simulink model "EPD629_WilliamsJ_AS12"  (R2021b)
settings: Solver=VariableStepAuto  StartTime=0.0  StopTime=45  MaxStep=0.0005  RelTol=1e-3
values from neighbouring files (symbols this model uses):
  AirMassFracO2 = 0.233    [EPD629_HW12_init.m]
  BPVAreaBreakpoints_pct = BPVAreaData_pct    [EPD629_HW12_init.m]
  BPVAreaData_pct = EGRValveAreaData_pct    [EPD629_HW12_init.m]
  BPVPositionBreakpoints_pct = EGRValvePositionBreakpoints_pct    [EPD629_HW12_init.m]
  BPVPositionData_pct = BPVPositionBreakpoints_pct    [EPD629_HW12_init.m]
  BPVWideOpenArea_mm2 = pi * BPVDiameter_mm^2 / 4    (= 7853.98163397)    [EPD629_HW12_init.m]
  CACDischargeCoefficient_frac = 0.7    [EPD629_HW12_init.m]
  CACEffectivenessData_frac = [1 0.95 0.92 0.885 0.87 0.85]    [EPD629_HW12_init.m]
  CACEffectivenessMassFlowBP_gps = [0 50 100 200 300 500]    [EPD629_HW12_init.m]
  CACFlowRestrictionArea_mm2 = 2000    [EPD629_HW12_init.m]
  CACVolume_L = 40    [EPD629_HW12_init.m]
  ClearanceVolumeTotal_L = 8/15    (= 0.533333333333)    [EPD629_HW12_init.m]
  Cp_cmp = 1.004    [EPD629_HW12_init.m]
  Cp_trb = 1.073    [EPD629_HW12_init.m]
  DesiredFuelBreakpoints_mg = 0:20:500    [EPD629_HW12_init.m]
  DischargeCoefficient_frac = 0.7    [EPD629_HW12_init.m]
  EGRCDischargeCoefficient_frac = 0.7    [EPD629_HW12_init.m]
  EGRCEffectivenessData_frac = [1 0.95 0.92 0.885 0.87 0.85]    [EPD629_HW12_init.m]
  EGRCEffectivenessMassFlowBP_gps = [0 50 100 200 300 500]    [EPD629_HW12_init.m]
  EGRCFlowRestrictionArea_mm2 = 500    [EPD629_HW12_init.m]
  EGRCoolerToValveVolume_L = 2    [EPD629_HW12_init.m]
  EGRValveAreaBreakpoints_pct = EGRValveAreaData_pct    [EPD629_HW12_init.m]
  EGRValveAreaData_pct = 100 * EGRValveArea_mm2 / EGRValveWideOpenArea_mm2    [EPD629_HW12_init.m]
  EGRValvePositionBreakpoints_pct = 0:100    [EPD629_HW12_init.m]
  EGRValvePositionData_pct = EGRValvePositionBreakpoints_pct    [EPD629_HW12_init.m]
  EGRValveWideOpenArea_mm2 = pi/4*50^2    (= 1963.49540849)    [EPD629_HW12_init.m]
  EngineDisplacement_L = 8    [EPD629_HW12_init.m]
  EngineSpeedBreakpoints_rpm = 600:200:3000    [EPD629_HW12_init.m]
  ExhaustManifoldGasConstant_kJpkgK = R_trb    (= 0.287)    [EPD629_HW12_init.m]
  ExhaustManifoldVolume_L = 8    [EPD629_HW12_init.m]
  FlowFunctionData_frac = PR.^(1/k_trb) .*      sqrt( 2 * k_trb / (k_trb - 1) .*      (1 - PR.^((k_trb - 1) / k_trb)) )    [EPD629_HW12_init.m]
  IntakeManifoldGasConstant_kJpkgK = Cp_im - Cv_im    (= 0.288)    [EPD629_HW12_init.m]
  IntakeManifoldVolume_L = 8    [EPD629_HW12_init.m]
  k_cmp = Cp_cmp/Cv_cmp    (= 1.40027894003)    [EPD629_HW12_init.m]
  k_trb = Cp_trb/Cv_trb    (= 1.36513994911)    [EPD629_HW12_init.m]
  ManifoldPressureBreakpoints_kPa = 80:20:500    [EPD629_HW12_init.m]
  NumberOfCylinders = 6    [EPD629_HW12_init.m]
  PressureRatioBreakpoints_frac = 0:0.01:1    [EPD629_HW12_init.m]
  R_cmp = Cp_cmp - Cv_cmp    (= 0.287)    [EPD629_HW12_init.m]
  R_trb = Cp_trb - Cv_trb    (= 0.287)    [EPD629_HW12_init.m]
  StoichiometricAFR_frac = 14.7    [EPD629_HW12_init.m]
  TurbineToBPVVolume_L = 10    [EPD629_HW12_init.m]
  TurbochargerInertia_kgm2 = 1e-4    (= 0.0001)    [EPD629_HW12_init.m]
  WastegateAreaData_pct = [0 100]    [EPD629_HW12_init.m]
  WastegateAreaGagePressBreakpoints_kPa = [250 300]    [EPD629_HW12_init.m]
  WastegateWideOpenArea_mm2 = pi/4*20^2    (= 314.159265359)    [EPD629_HW12_init.m]
undefined symbols (not defined in the file or in its folder): APPR_cmp, APPR_trb, ARPM_cmp, ARPM_trb, EFFI_cmp, EFFI_trb, ExhaustTemperatureData_degC, MASS_cmp, MASS_trb, MXRSP_cmp, MXRSP_trb, MXRVOL_cmp, MXRVOL_trb, PMAX_cmp, PMAX_trb, PMIN_cmp, PMIN_trb, ResidualCorrectionFactorData, VolumetricEfficiencyData_frac
libraries: simulink x2
(part 1 of 3)
settings Model: Creator=John  LastModifiedBy=Justin
settings SolverCC: AlgebraicLoopSolver=TrustRegion
settings DebuggingCC: SFMachineParentedDataDiag=warning

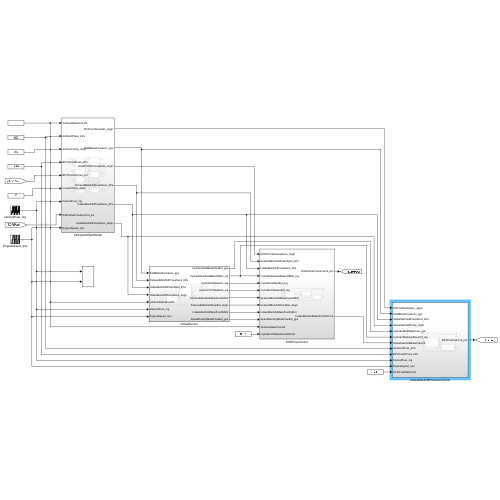
[thumbnail: Simulink's stored preview of the top-level diagram]
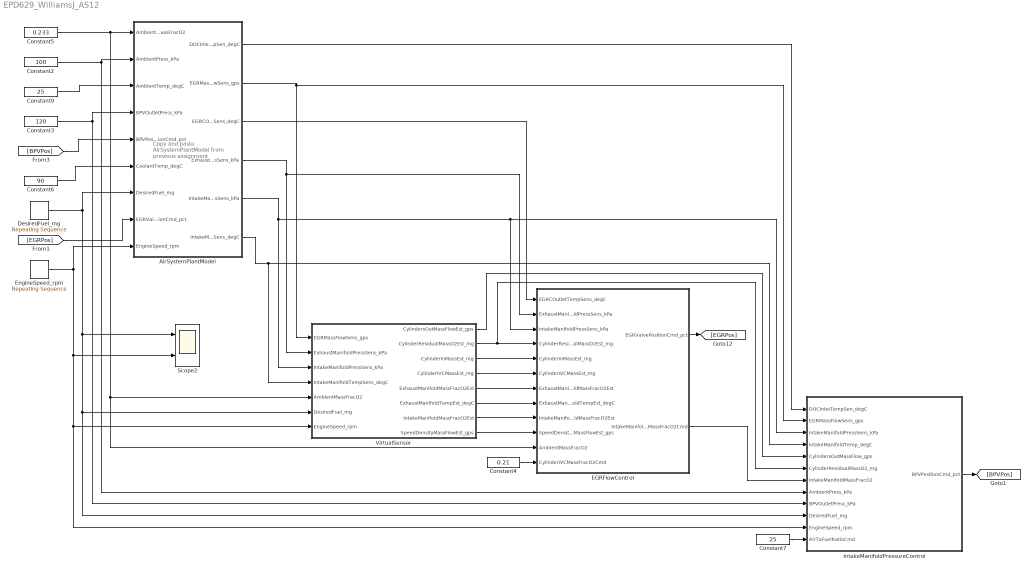
== system EPD629_WilliamsJ_AS12 ==
  note: Copy and paste
      | AirSystemPlantModel
      | from previous assignment
  AirSystemPlantModel : Subsystem
  Constant2 : Constant  Value=100
  Constant3 : Constant  Value=120
  Constant4 : Constant  Value=0.21
  Constant5 : Constant  Value=0.233
  Constant6 : Constant  Value=90
  Constant7 : Constant  Value=25
  Constant9 : Constant  Value=25
  DesiredFuel_mg : simulink/Sources/Repeating Sequence  rep_seq_t="0.25*[0 20 20.1 40 40.1 60    60.1 80 80.1 100 100.1 120    120.1 140 140.1 160 160.1 180]"  rep_seq_y="[40 40 80 80 120 120    70 70 140 140 210 210    90 90 180 180 220 220]"
  EGRFlowControl : Subsystem
  EngineSpeed_rpm : simulink/Sources/Repeating Sequence  rep_seq_t=0.25*[0 60 60.1 120 120.1 180]  rep_seq_y=[1200 1200 1600 1600 2000 2000]
  IntakeManifoldPressureControl : Subsystem
  Scope2 : Scope  NumInputPorts=2
  VirtualSensor : Subsystem
  wires:
  Constant9/1 -> AirSystemPlantModel/3(AmbientTemp_degC)
  Constant6/1 -> AirSystemPlantModel/6(CoolantTemp_degC)
  Constant2/1 -> AirSystemPlantModel/2(AmbientPress_kPa), IntakeManifoldPressureControl/8(AmbientPress_kPa)
  Constant3/1 -> AirSystemPlantModel/4(BPVOutletPress_kPa), IntakeManifoldPressureControl/9(BPVOutletPress_kPa)
  [BPVPos] -> AirSystemPlantModel/5(BPVPositionCmd_pct)
  Constant5/1 -> AirSystemPlantModel/1(AmbientMassFracO2), VirtualSensor/5(AmbientMassFracO2), EGRFlowControl/11(AmbientMassFracO2)
  AirSystemPlantModel/2(EGRMassFlowSens_gps) -> VirtualSensor/1(EGRMassFlowSens_gps), IntakeManifoldPressureControl/2(EGRMassFlowSens_gps)
  AirSystemPlantModel/4(ExhaustManifoldPressSens_kPa) -> VirtualSensor/2(ExhaustManifoldPressSens_kPa), EGRFlowControl/2(ExhaustManifoldPressSens_kPa)
  AirSystemPlantModel/5(IntakeManifoldPressSens_kPa) -> EGRFlowControl/3(IntakeManifoldPressSens_kPa), IntakeManifoldPressureControl/3(IntakeManifoldPressSens_kPa), VirtualSensor/3(IntakeManifoldPressSens_kPa)
  AirSystemPlantModel/6(IntakeManifoldTempSens_degC) -> VirtualSensor/4(IntakeManifoldTempSens_degC), IntakeManifoldPressureControl/4(IntakeManifoldTemp_degC)
  VirtualSensor/5(ExhaustManifoldMassFracO2Est) -> EGRFlowControl/7(ExhaustManifoldMassFracO2Est)
  VirtualSensor/7(IntakeManifoldMassFracO2Est) -> EGRFlowControl/9(IntakeManifoldMassFracO2Est)
  VirtualSensor/3(CylinderInMassEst_mg) -> EGRFlowControl/5(CylinderInMassEst_mg)
  VirtualSensor/4(CylinderIVCMassEst_mg) -> EGRFlowControl/6(CylinderIVCMassEst_mg)
  Constant4/1 -> EGRFlowControl/12(CylinderIVCMassFracO2Cmd)
  DesiredFuel_mg/1 -> AirSystemPlantModel/7(DesiredFuel_mg), IntakeManifoldPressureControl/10(DesiredFuel_mg), VirtualSensor/6(DesiredFuel_mg), Scope2/1
  EngineSpeed_rpm/1 -> AirSystemPlantModel/9(EngineSpeed_rpm), IntakeManifoldPressureControl/11(EngineSpeed_rpm), VirtualSensor/7(EngineSpeed_rpm), Scope2/2
  VirtualSensor/2(CylinderResidualMassO2Est_mg) -> EGRFlowControl/4(CylinderResidualMassO2Est_mg), IntakeManifoldPressureControl/6(CylinderResidualMassO2_mg)
  EGRFlowControl/2(IntakeManifoldMassFracO2Cmd) -> IntakeManifoldPressureControl/7(IntakeManifoldMassFracO2)
  Constant7/1 -> IntakeManifoldPressureControl/12(AirToFuelRatioCmd)
  [EGRPos] -> AirSystemPlantModel/8(EGRValvePositionCmd_pct)
  AirSystemPlantModel/1(DOCInletTempSen_degC) -> IntakeManifoldPressureControl/1(DOCInletTempSen_degC)
  VirtualSensor/8(SpeedDensityMassFlowEst_gps) -> EGRFlowControl/10(SpeedDensityMassFlowEst_gps)
  EGRFlowControl/1(EGRValvePositionCmd_pct) -> [EGRPos]
  AirSystemPlantModel/3(EGRCOutletTempSens_degC) -> EGRFlowControl/1(EGRCOutletTempSens_degC)
  VirtualSensor/6(ExhaustManifoldTempEst_degC) -> EGRFlowControl/8(ExhaustManifoldTempEst_degC)
  IntakeManifoldPressureControl/1(BPVPositionCmd_pct) -> [BPVPos]
  VirtualSensor/1(CylindersOutMassFlowEst_gps) -> IntakeManifoldPressureControl/5(CylindersOutMassFlow_gps)

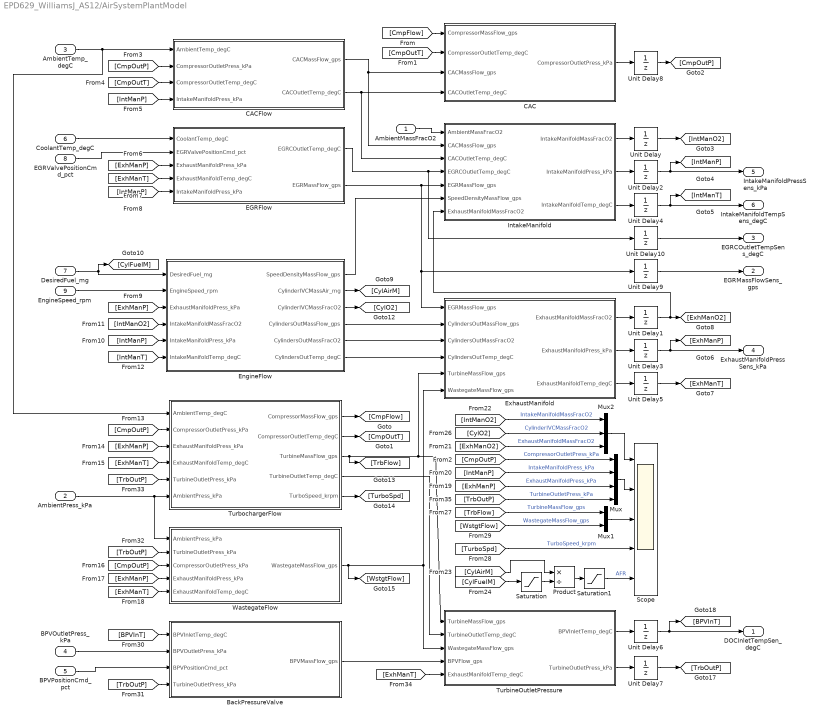
== system EPD629_WilliamsJ_AS12/AirSystemPlantModel ==
  AmbientMassFracO2 : Inport
  AmbientPress_kPa : Inport  Port=2
  AmbientTemp_degC : Inport  Port=3
  BPVOutletPress_kPa : Inport  Port=4
  BPVPositionCmd_pct : Inport  Port=5
  CoolantTemp_degC : Inport  Port=6
  DesiredFuel_mg : Inport  Port=7
  EGRValvePositionCmd_pct : Inport  Port=8
  EngineSpeed_rpm : Inport  Port=9
  BackPressureValve : Subsystem
  CAC : Subsystem
  CACFlow : Subsystem
  EGRFlow : Subsystem
  EngineFlow : Subsystem
  ExhaustManifold : Subsystem
  IntakeManifold : Subsystem
  Mux : Mux
  Mux1 : Mux  Inputs=2
  Mux2 : Mux  Inputs=3
  Product : Product  Inputs=*/
  Saturation : Saturate  UpperLimit=1000  LowerLimit=0.1
  Saturation1 : Saturate  UpperLimit=200  LowerLimit=0
  Scope : Scope  NumInputPorts=5
  TurbineOutletPressure : Subsystem
  TurbochargerFlow : Subsystem
  Unit Delay : UnitDelay  InitialCondition=0.233  SampleTime=-1  HasFrameUpgradeWarning=on
      settings: AttributesFormatString=IC: %<InitialCondition>
  Unit Delay1 : UnitDelay  InitialCondition=0.233  SampleTime=-1  HasFrameUpgradeWarning=on
      settings: AttributesFormatString=IC: %<InitialCondition>
  Unit Delay{4..6,10} (4 alike) : UnitDelay  InitialCondition=25  SampleTime=-1  HasFrameUpgradeWarning=on
      settings: AttributesFormatString=IC: %<InitialCondition>
  Unit Delay{2..3,7..8} (4 alike) : UnitDelay  InitialCondition=100  SampleTime=-1  HasFrameUpgradeWarning=on
      settings: AttributesFormatString=IC: %<InitialCondition>
  Unit Delay9 : UnitDelay  SampleTime=-1  HasFrameUpgradeWarning=on
      settings: AttributesFormatString=IC: %<InitialCondition>
  WastegateFlow : Subsystem
  DOCInletTempSen_degC : Outport
  EGRMassFlowSens_gps : Outport  Port=2
  EGRCOutletTempSens_degC : Outport  Port=3
  ExhaustManifoldPressSens_kPa : Outport  Port=4
  IntakeManifoldPressSens_kPa : Outport  Port=5
  IntakeManifoldTempSens_degC : Outport  Port=6
  wires:
  [IntManT] -> EngineFlow/6(IntakeManifoldTemp_degC)
  AmbientPress_kPa/1 -> WastegateFlow/1(AmbientPress_kPa), TurbochargerFlow/6(AmbientPress_kPa)
  [ExhManO2] -> Mux2/3  "ExhaustManifoldMassFracO2"
  [ExhManP] -> Mux/3  "ExhaustManifoldPress_kPa"
  EGRFlow/2(EGRMassFlow_gps) -> ExhaustManifold/1(EGRMassFlow_gps), Unit Delay9/1, IntakeManifold/5(EGRMassFlow_gps)
  Mux/1 -> Scope/2
  [CmpOutT] -> CAC/2(CompressorOutletTemp_degC)
  [ExhManP] -> EngineFlow/3(ExhaustManifoldPress_kPa)
  AmbientTemp_degC/1 -> TurbochargerFlow/1(AmbientTemp_degC), CACFlow/1(AmbientTemp_degC)
  [TrbFlow] -> Mux1/1  "TurbineMassFlow_gps"
  ExhaustManifold/3(ExhaustManifoldTemp_degC) -> Unit Delay5/1
  CACFlow/1(CACMassFlow_gps) -> IntakeManifold/2(CACMassFlow_gps), CAC/3(CACMassFlow_gps)
  [ExhManP] -> TurbochargerFlow/3(ExhaustManifoldPress_kPa)
  EGRValvePositionCmd_pct/1 -> EGRFlow/2(EGRValvePositionCmd_pct)
  [CmpOutP] -> TurbochargerFlow/2(CompressorOutletPress_kPa)
  TurbochargerFlow/2(CompressorOutletTemp_degC) -> [CmpOutT]
  [TurboSpd] -> Scope/4  "TurboSpeed_krpm"
  [CmpOutP] -> CACFlow/2(CompressorOutletPress_kPa)
  [CmpOutT] -> CACFlow/3(CompressorOutletTemp_degC)
  CACFlow/2(CACOutletTemp_degC) -> CAC/4(CACOutletTemp_degC), IntakeManifold/3(CACOutletTemp_degC)
  [IntManP] -> CACFlow/4(IntakeManifoldPress_kPa)
  [BPVInT] -> BackPressureValve/1(BPVInletTemp_degC)
  EngineSpeed_rpm/1 -> EngineFlow/2(EngineSpeed_rpm)
  WastegateFlow/1(WastegateMassFlow_gps) -> ExhaustManifold/6(WastegateMassFlow_gps), TurbineOutletPressure/3(WastegateMassFlow_gps), [WstgtFlow]
  CAC/1(CompressorOutletPress_kPa) -> Unit Delay8/1
  Mux1/1 -> Scope/3
  TurbochargerFlow/5(TurboSpeed_krpm) -> [TurboSpd]
  TurbochargerFlow/1(CompressorMassFlow_gps) -> [CmpFlow]
  [ExhManT] -> WastegateFlow/5(ExhaustManifoldTemp_degC)
  [IntManO2] -> EngineFlow/4(IntakeManifoldMassFracO2)
  [ExhManP] -> WastegateFlow/4(ExhaustManifoldPress_kPa)
  [CmpFlow] -> CAC/1(CompressorMassFlow_gps)
  [ExhManT] -> TurbochargerFlow/4(ExhaustManifoldTemp_degC)
  DesiredFuel_mg/1 -> [CylFuelM], EngineFlow/1(DesiredFuel_mg)
  [CmpOutP] -> WastegateFlow/3(CompressorOutletPress_kPa)
  TurbochargerFlow/3(TurbineMassFlow_gps) -> [TrbFlow], ExhaustManifold/5(TurbineMassFlow_gps), TurbineOutletPressure/1(TurbineMassFlow_gps)
  [ExhManP] -> EGRFlow/3(ExhaustManifoldPress_kPa)
  IntakeManifold/3(IntakeManifoldTemp_degC) -> Unit Delay4/1
  BackPressureValve/1(BPVMassFlow_gps) -> TurbineOutletPressure/4(BPVFlow_gps)
  [IntManP] -> EGRFlow/5(IntakeManifoldPress_kPa)
  [CmpOutP] -> Mux/1  "CompressorOutletPress_kPa"
  EngineFlow/1(SpeedDensityMassFlow_gps) -> IntakeManifold/6(SpeedDensityMassFlow_gps)
  ExhaustManifold/2(ExhaustManifoldPress_kPa) -> Unit Delay3/1
  IntakeManifold/2(IntakeManifoldPress_kPa) -> Unit Delay2/1
  EGRFlow/1(EGRCOutletTemp_degC) -> Unit Delay10/1, IntakeManifold/4(EGRCOutletTemp_degC)
  Mux2/1 -> Scope/1
  TurbochargerFlow/4(TurbineOutletTemp_degC) -> TurbineOutletPressure/2(TurbineOutletTemp_degC)
  [IntManO2] -> Mux2/1  "IntakeManifoldMassFracO2"
  [IntManP] -> Mux/2  "IntakeManifoldPress_kPa"
  [TrbOutP] -> Mux/4  "TurbineOutletPress_kPa"
  [ExhManT] -> EGRFlow/4(ExhaustManifoldTemp_degC)
  [CylO2] -> Mux2/2  "CylinderIVCMassFracO2"
  [WstgtFlow] -> Mux1/2  "WastegateMassFlow_gps"
  TurbineOutletPressure/1(BPVInletTemp_degC) -> Unit Delay6/1
  [TrbOutP] -> BackPressureValve/4(TurbineOutletPress_kPa)
  TurbineOutletPressure/2(TurbineOutletPress_kPa) -> Unit Delay7/1
  [TrbOutP] -> TurbochargerFlow/5(TurbineOutletPress_kPa)
  [TrbOutP] -> WastegateFlow/2(TurbineOutletPress_kPa)
  [ExhManT] -> TurbineOutletPressure/5(ExhaustManifoldTemp_degC)
  CoolantTemp_degC/1 -> EGRFlow/1(CoolantTemp_degC)
  BPVOutletPress_kPa/1 -> BackPressureValve/2(BPVOutletPress_kPa)
  BPVPositionCmd_pct/1 -> BackPressureValve/3(BPVPositionCmd_pct)
  AmbientMassFracO2/1 -> IntakeManifold/1(AmbientMassFracO2)
  IntakeManifold/1(IntakeManifoldMassFracO2) -> Unit Delay/1
  Unit Delay/1 -> [IntManO2]
  Unit Delay1/1 -> IntakeManifold/7(ExhaustManifoldMassFracO2), [ExhManO2]
  Unit Delay2/1 -> IntakeManifoldPressSens_kPa/1, [IntManP]
  Unit Delay3/1 -> ExhaustManifoldPressSens_kPa/1, [ExhManP]
  Unit Delay4/1 -> IntakeManifoldTempSens_degC/1, [IntManT]
  Unit Delay5/1 -> [ExhManT]
  Unit Delay6/1 -> [BPVInT], DOCInletTempSen_degC/1
  Unit Delay7/1 -> [TrbOutP]
  Unit Delay8/1 -> [CmpOutP]
  Unit Delay9/1 -> EGRMassFlowSens_gps/1
  ExhaustManifold/1(ExhaustManifoldMassFracO2) -> Unit Delay1/1
  Unit Delay10/1 -> EGRCOutletTempSens_degC/1
  Product/1 -> Saturation1/1
  [CylFuelM] -> Saturation/1
  Saturation/1 -> Product/2
  [CylAirM] -> Product/1
  Saturation1/1 -> Scope/5  "AFR"
  [IntManP] -> EngineFlow/5(IntakeManifoldPress_kPa)
  EngineFlow/6(CylindersOutTemp_degC) -> ExhaustManifold/4(CylindersOutTemp_degC)
  EngineFlow/5(CylindersOutMassFracO2) -> ExhaustManifold/3(CylindersOutMassFracO2)
  EngineFlow/4(CylindersOutMassFlow_gps) -> ExhaustManifold/2(CylindersOutMassFlow_gps)
  EngineFlow/2(CylinderIVCMassAir_mg) -> [CylAirM]
  EngineFlow/3(CylinderIVCMassFracO2) -> [CylO2]

== system EPD629_WilliamsJ_AS12/EGRFlowControl ==
  EGRCOutletTempSens_degC : Inport
  ExhaustManifoldPressSens_kPa : Inport  Port=2
  IntakeManifoldPressSens_kPa : Inport  Port=3
  CylinderResidualMassO2Est_mg : Inport  Port=4
  CylinderInMassEst_mg : Inport  Port=5
  CylinderIVCMassEst_mg : Inport  Port=6
  ExhaustManifoldMassFracO2Est : Inport  Port=7
  ExhaustManifoldTempEst_degC : Inport  Port=8
  IntakeManifoldMassFracO2Est : Inport  Port=9
  SpeedDensityMassFlowEst_gps : Inport  Port=10
  AmbientMassFracO2 : Inport  Port=11
  CylinderIVCMassFracO2Cmd : Inport  Port=12
  CoolerOutletPressureCommand : Subsystem
  EGRMassFlowCommand : Subsystem
  EGRValvePositionCommand : Subsystem
  IntakeManifoldMassFractionO2Command : Subsystem
  Mux : Mux  Inputs=2
  Scope2 : Scope  NumInputPorts=4
  EGRValvePositionCmd_pct : Outport
  IntakeManifoldMassFracO2Cmd : Outport  Port=2
  wires:
  CylinderInMassEst_mg/1 -> IntakeManifoldMassFractionO2Command/1(CylinderInMassEst_mg)
  CylinderIVCMassEst_mg/1 -> IntakeManifoldMassFractionO2Command/2(CylinderIVCMassEst_mg)
  CylinderIVCMassFracO2Cmd/1 -> IntakeManifoldMassFractionO2Command/3(CylinderIVCMassFracO2Cmd)
  EGRValvePositionCommand/1(EGRValvePositionCmd_pct) -> EGRMassFlowCommand/6(EGRValvePositionCmd_pct), Scope2/4, EGRValvePositionCmd_pct/1
  IntakeManifoldMassFracO2Est/1 -> Mux/2, EGRMassFlowCommand/2(IntakeManifoldMassFracO2Est)
  AmbientMassFracO2/1 -> EGRMassFlowCommand/3(AmbientMassFracO2)
  SpeedDensityMassFlowEst_gps/1 -> EGRMassFlowCommand/5(SpeedDensityMassFlowEst_gps)
  ExhaustManifoldMassFracO2Est/1 -> EGRMassFlowCommand/4(ExhaustManifoldMassFracO2Est)
  IntakeManifoldMassFractionO2Command/1(IntakeManifoldMassFracO2Cmd) -> IntakeManifoldMassFracO2Cmd/1, EGRMassFlowCommand/1(IntakeManifoldMassFracO2Cmd), Mux/1
  CylinderResidualMassO2Est_mg/1 -> IntakeManifoldMassFractionO2Command/4(CylinderResidualMassO2Est_mg)
  EGRCOutletTempSens_degC/1 -> EGRValvePositionCommand/2(EGRCOutletTempSens_degC), CoolerOutletPressureCommand/3(EGRCOutletTempSens_degC)
  ExhaustManifoldPressSens_kPa/1 -> CoolerOutletPressureCommand/1(ExhaustManifoldPressSens_kPa)
  IntakeManifoldPressSens_kPa/1 -> EGRValvePositionCommand/4(IntakeManifoldPressSens_kPa)
  CoolerOutletPressureCommand/1(EGRCOutletPressCmd_kPa) -> EGRValvePositionCommand/1(EGRCOutletPressCmd_kPa), Scope2/3
  EGRMassFlowCommand/1(EGRMassFlowCmd_gps) -> Scope2/2, CoolerOutletPressureCommand/4(EGRMassFlowCmd_gps), EGRValvePositionCommand/3(EGRMassFlowCmd_gps)
  ExhaustManifoldTempEst_degC/1 -> CoolerOutletPressureCommand/2(ExhaustManifoldTempEst_degC)
  Mux/1 -> Scope2/1

== system EPD629_WilliamsJ_AS12/IntakeManifoldPressureControl ==
  DOCInletTempSen_degC : Inport
  EGRMassFlowSens_gps : Inport  Port=2
  IntakeManifoldPressSens_kPa : Inport  Port=3
  IntakeManifoldTemp_degC : Inport  Port=4
  CylindersOutMassFlow_gps : Inport  Port=5
  CylinderResidualMassO2_mg : Inport  Port=6
  IntakeManifoldMassFracO2 : Inport  Port=7
  AmbientPress_kPa : Inport  Port=8
  BPVOutletPress_kPa : Inport  Port=9
  DesiredFuel_mg : Inport  Port=10
  EngineSpeed_rpm : Inport  Port=11
  AirToFuelRatioCmd : Inport  Port=12
  BPVInletPressureCommand : Subsystem
  BPVPositionCommand : Subsystem
  IntakeManifoldPressureCommand : Subsystem
  Mux : Mux  Inputs=2
  Scope2 : Scope  NumInputPorts=3
  BPVPositionCmd_pct : Outport
  wires:
  CylindersOutMassFlow_gps/1 -> BPVInletPressureCommand/4(CylindersOutMassFlow_gps)
  EGRMassFlowSens_gps/1 -> BPVInletPressureCommand/5(EGRMassFlowSens_gps)
  IntakeManifoldPressSens_kPa/1 -> Mux/2, BPVInletPressureCommand/3(IntakeManifoldPressSens_kPa)
  BPVInletPressureCommand/1(BPVMassFlowCmd_gps) -> BPVPositionCommand/1(BPVMassFlowCmd_gps)
  BPVInletPressureCommand/2(BPVInletPressCmd_kPa) -> Scope2/2, BPVPositionCommand/2(BPVInletPressCmd_kPa)
  IntakeManifoldTemp_degC/1 -> IntakeManifoldPressureCommand/1(IntakeManifoldTemp_degC)
  CylinderResidualMassO2_mg/1 -> IntakeManifoldPressureCommand/2(CylinderResidualMassO2_mg)
  IntakeManifoldMassFracO2/1 -> IntakeManifoldPressureCommand/3(IntakeManifoldMassFracO2)
  DesiredFuel_mg/1 -> IntakeManifoldPressureCommand/4(DesiredFuel_mg)
  EngineSpeed_rpm/1 -> IntakeManifoldPressureCommand/5(EngineSpeed_rpm)
  AirToFuelRatioCmd/1 -> IntakeManifoldPressureCommand/6(AirToFuelRatioCmd)
  IntakeManifoldPressureCommand/1(IntakeManifoldPressCmd_kPa) -> BPVInletPressureCommand/1(IntakeManifoldPressCmd_kPa), Mux/1
  BPVPositionCommand/1(BPVPositionCmd_pct) -> BPVInletPressureCommand/6(BPVPositionCmd_pct), Scope2/3, BPVPositionCmd_pct/1
  DOCInletTempSen_degC/1 -> BPVPositionCommand/4(DOCInletTempSen_degC)
  BPVOutletPress_kPa/1 -> BPVPositionCommand/3(BPVOutletPress_kPa)
  Mux/1 -> Scope2/1
  AmbientPress_kPa/1 -> BPVInletPressureCommand/2(AmbientPress_kPa), IntakeManifoldPressureCommand/7(AmbientPress_kPa)

== system EPD629_WilliamsJ_AS12/VirtualSensor ==
  EGRMassFlowSens_gps : Inport
  ExhaustManifoldPressSens_kPa : Inport  Port=2
  IntakeManifoldPressSens_kPa : Inport  Port=3
  IntakeManifoldTempSens_degC : Inport  Port=4
  AmbientMassFracO2 : Inport  Port=5
  DesiredFuel_mg : Inport  Port=6
  EngineSpeed_rpm : Inport  Port=7
  EngineFlow : Subsystem
  ExhaustManifoldMassFraction : Subsystem
  IntakeManifoldMassFraction : Subsystem
  Terminator : Terminator
  Terminator1 : Terminator
  Terminator2 : Terminator
  CylindersOutMassFlowEst_gps : Outport
  CylinderResidualMassO2Est_mg : Outport  Port=2
  CylinderInMassEst_mg : Outport  Port=3
  CylinderIVCMassEst_mg : Outport  Port=4
  ExhaustManifoldMassFracO2Est : Outport  Port=5
  ExhaustManifoldTempEst_degC : Outport  Port=6
  IntakeManifoldMassFracO2Est : Outport  Port=7
  SpeedDensityMassFlowEst_gps : Outport  Port=8
  wires:
  EngineFlow/10(SpeedDensityMassFlow_gps) -> SpeedDensityMassFlowEst_gps/1, IntakeManifoldMassFraction/6(SpeedDensityMassFlowEst_gps)
  DesiredFuel_mg/1 -> EngineFlow/2(DesiredFuel_mg)
  EngineSpeed_rpm/1 -> EngineFlow/3(EngineSpeed_rpm)
  AmbientMassFracO2/1 -> IntakeManifoldMassFraction/3(AmbientMassFracO2)
  EGRMassFlowSens_gps/1 -> IntakeManifoldMassFraction/4(EGRMassFlowSens_gps)
  IntakeManifoldMassFraction/1(IntakeManifoldMassFracO2Est) -> EngineFlow/6(IntakeManifoldMassFracO2), IntakeManifoldMassFracO2Est/1
  IntakeManifoldPressSens_kPa/1 -> IntakeManifoldMassFraction/1(IntakeManifoldPressSens_kPa), EngineFlow/4(IntakeManifoldPress_kPa)
  IntakeManifoldTempSens_degC/1 -> IntakeManifoldMassFraction/2(IntakeManifoldTemp_degC), EngineFlow/5(IntakeManifoldTemp_degC)
  ExhaustManifoldPressSens_kPa/1 -> EngineFlow/1(ExhaustManifoldPress_kPa), ExhaustManifoldMassFraction/1(ExhaustManifoldPressSens_kPa)
  EngineFlow/1(CylindersOutMassFlow_gps) -> ExhaustManifoldMassFraction/2(CylindersOutMassFlowEst_gps), CylindersOutMassFlowEst_gps/1
  EngineFlow/3(CylindersOutTemp_degC) -> ExhaustManifoldTempEst_degC/1, ExhaustManifoldMassFraction/4(CylindersOutTempEst_degC)
  EngineFlow/2(CylindersOutMassFracO2) -> ExhaustManifoldMassFraction/3(CylindersOutMassFracO2Est)
  ExhaustManifoldMassFraction/1(ExhaustManifoldMassFracO2Est) -> IntakeManifoldMassFraction/5(ExhaustManifoldMassFracO2Est), ExhaustManifoldMassFracO2Est/1
  EngineFlow/4(CylinderInMass_mg) -> CylinderInMassEst_mg/1
  EngineFlow/6(CylinderIVCMassAir_mg) -> Terminator/1
  EngineFlow/7(CylinderIVCMassFracO2) -> Terminator1/1
  EngineFlow/5(CylinderIVCMass_mg) -> CylinderIVCMassEst_mg/1
  EngineFlow/9(CylinderResidualMassO2_mg) -> CylinderResidualMassO2Est_mg/1
  EngineFlow/8(CylinderResidualMass_mg) -> Terminator2/1

== system EPD629_WilliamsJ_AS12/AirSystemPlantModel/BackPressureValve ==
  note: K
  note: g*m/s^2/mm^2
  note: m^2/s^2
  note: k kg*m/s^2/m^2
  note: N*m/kg
  note: m/s
  note: kPa
  BPVInletTemp_degC : Inport
  BPVOutletPress_kPa : Inport  Port=2
  BPVPositionCmd_pct : Inport  Port=3
  TurbineOutletPress_kPa : Inport  Port=4
  Add1 : Sum
  BPVAreaData_pct Table : Lookup_n-D  NumberOfTableDimensions=1  BreakpointsForDimension1=BPVPositionBreakpoints_pct  Table=BPVAreaData_pct  ExtrapMethod=Clip  UseLastTableValue=on  InternalRulePriority=Speed  RndMeth=Simplest  InputSameDT=on
  Constant : Constant  Value=273.15
  Constant1 : Constant  Value=DischargeCoefficient_frac
  Constant2 : Constant
  Constant3 : Constant  Value=ExhaustManifoldGasConstant_kJpkgK
  Constant5 : Constant  Value=BPVWideOpenArea_mm2
  Constant6 : Constant  Value=100
  FlowFunctionData_frac Table : Lookup_n-D  NumberOfTableDimensions=1  BreakpointsForDimension1=PressureRatioBreakpoints_frac  Table=FlowFunctionData_frac  ExtrapMethod=Clip  UseLastTableValue=on  InternalRulePriority=Speed  RndMeth=Simplest  InputSameDT=on
  Math Function : Math  Operator=sqrt  SignedPower=on  SaturateOnIntegerOverflow=on
  Max2 : MinMax  Function=max  Inputs=2
  Product : Product  Inputs=**/
  Product1 : Product  Inputs=****/  SaturateOnIntegerOverflow=on  OutDataTypeStr=Inherit: Same as first input
  Product2 : Product  Inputs=*/  SaturateOnIntegerOverflow=on  OutDataTypeStr=Inherit: Same as first input
  Product3 : Product  SaturateOnIntegerOverflow=on  OutDataTypeStr=Inherit: Same as first input
  Transfer Fcn : TransferFcn  Denominator=[0.05 1]
  kJ/(kg*K) to J/(kg*K) : Gain  Gain=1000
  BPVMassFlow_gps : Outport
  wires:
  Add1/1 -> Max2/1
  Constant/1 -> Add1/2
  Constant2/1 -> Max2/2
  BPVInletTemp_degC/1 -> Add1/1
  BPVPositionCmd_pct/1 -> Transfer Fcn/1
  Product/1 -> Product1/1  "BPVArea_mm2"
  Constant5/1 -> Product/2
  Constant6/1 -> Product/3
  Product3/1 -> Math Function/1
  Math Function/1 -> Product1/5
  Max2/1 -> Product3/2
  kJ/(kg*K) to J/(kg*K)/1 -> Product3/1
  Constant3/1 -> kJ/(kg*K) to J/(kg*K)/1
  Constant1/1 -> Product1/2
  Product2/1 -> FlowFunctionData_frac Table/1  "BPVPressureRatio_frac"
  FlowFunctionData_frac Table/1 -> Product1/3
  BPVAreaData_pct Table/1 -> Product/1  "BPVArea_pct"
  TurbineOutletPress_kPa/1 -> Product2/2, Product1/4
  Product1/1 -> BPVMassFlow_gps/1
  BPVOutletPress_kPa/1 -> Product2/1
  Transfer Fcn/1 -> BPVAreaData_pct Table/1

== system EPD629_WilliamsJ_AS12/AirSystemPlantModel/CAC ==
  note: dm/dt
  note: dP/dt
  CompressorMassFlow_gps : Inport
  CompressorOutletTemp_degC : Inport  Port=2
  CACMassFlow_gps : Inport  Port=3
  CACOutletTemp_degC : Inport  Port=4
  Add : Sum  Inputs=+-
  Add1 : Sum  Inputs=2
  Add2 : Sum
  Constant : Constant  Value=273.15
  Constant2 : Constant  Value=IntakeManifoldGasConstant_kJpkgK
  Constant3 : Constant  Value=CACVolume_L
  Gain : Gain  Gain=0.5
  Integrator3 : Integrator  InitialCondition=100  LimitOutput=on  UpperSaturationLimit=1000  LowerSaturationLimit=10
      settings: AttributesFormatString=|
      | Max: %<UpperSaturationLimit>
      | Min: %<LowerSaturationLimit>
      | IC: %<InitialCondition>
  Product1 : Product  Inputs=***/  RndMeth=Zero
  Saturation : Saturate  UpperLimit=1000  LowerLimit=-100
      settings: AttributesFormatString=|
      | Max: %<UpperLimit>
      | Min: %<LowerLimit>
  CompressorOutletPress_kPa : Outport
  wires:
  Constant3/1 -> Product1/4
  Constant2/1 -> Product1/2
  CACMassFlow_gps/1 -> Add/2
  CompressorMassFlow_gps/1 -> Add/1
  Add/1 -> Product1/1
  CompressorOutletTemp_degC/1 -> Add1/1
  CACOutletTemp_degC/1 -> Add1/2
  Add1/1 -> Gain/1
  Constant/1 -> Add2/2
  Gain/1 -> Saturation/1
  Add2/1 -> Product1/3
  Integrator3/1 -> CompressorOutletPress_kPa/1
  Product1/1 -> Integrator3/1
  Saturation/1 -> Add2/1

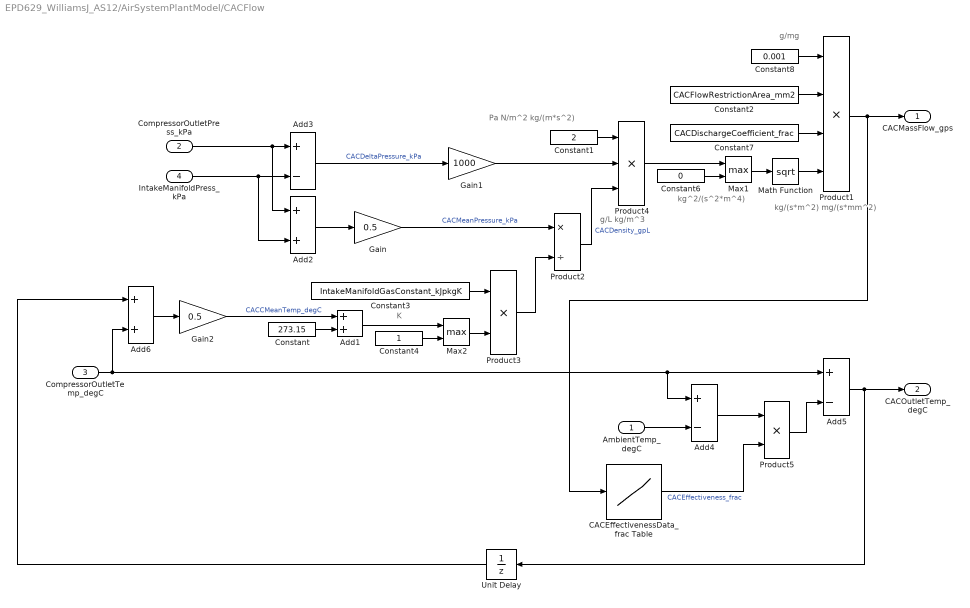
== system EPD629_WilliamsJ_AS12/AirSystemPlantModel/CACFlow ==
  note: g/mg
  note: g/L
      | kg/m^3
  note: kg^2/(s^2*m^4)
  note: Pa
      | N/m^2
      | kg/(m*s^2)
  note: K
  note: kg/(s*m^2)
      | mg/(s*mm^2)
  AmbientTemp_degC : Inport
  CompressorOutletPress_kPa : Inport  Port=2
  CompressorOutletTemp_degC : Inport  Port=3
  IntakeManifoldPress_kPa : Inport  Port=4
  Add1 : Sum
  Add2 : Sum  Inputs=2
  Add3 : Sum  Inputs=+-
  Add4 : Sum  Inputs=+-
  Add5 : Sum  Inputs=+-
  Add6 : Sum  Inputs=2
  CACEffectivenessData_frac Table : Lookup_n-D  NumberOfTableDimensions=1  BreakpointsForDimension1=CACEffectivenessMassFlowBP_gps  Table=CACEffectivenessData_frac  ExtrapMethod=Clip  UseLastTableValue=on  InternalRulePriority=Speed  RndMeth=Simplest  InputSameDT=on
  Constant : Constant  Value=273.15
  Constant1 : Constant  Value=2
  Constant2 : Constant  Value=CACFlowRestrictionArea_mm2
  Constant3 : Constant  Value=IntakeManifoldGasConstant_kJpkgK
  Constant4 : Constant
  Constant6 : Constant  Value=0
  Constant7 : Constant  Value=CACDischargeCoefficient_frac
  Constant8 : Constant  Value=0.001
  Gain : Gain  Gain=0.5
  Gain1 : Gain  Gain=1000
  Gain2 : Gain  Gain=0.5
  Math Function : Math  Operator=sqrt  SignedPower=on  SaturateOnIntegerOverflow=on
  Max1 : MinMax  Function=max  Inputs=2
  Max2 : MinMax  Function=max  Inputs=2
  Product1 : Product  Inputs=4  SaturateOnIntegerOverflow=on  OutDataTypeStr=Inherit: Same as first input
  Product2 : Product  Inputs=*/  SaturateOnIntegerOverflow=on  OutDataTypeStr=Inherit: Same as first input
  Product3 : Product  SaturateOnIntegerOverflow=on  OutDataTypeStr=Inherit: Same as first input
  Product4 : Product  Inputs=3  SaturateOnIntegerOverflow=on  OutDataTypeStr=Inherit: Same as first input
  Product5 : Product  SaturateOnIntegerOverflow=on  OutDataTypeStr=Inherit: Same as first input
  Unit Delay : UnitDelay  InitialCondition=100  SampleTime=-1  HasFrameUpgradeWarning=on
      settings: AttributesFormatString=IC: %<InitialCondition>
  CACMassFlow_gps : Outport
  CACOutletTemp_degC : Outport  Port=2
  wires:
  Constant2/1 -> Product1/2
  Constant3/1 -> Product3/1
  IntakeManifoldPress_kPa/1 -> Add3/2, Add2/2
  Add1/1 -> Max2/1
  Constant/1 -> Add1/2
  Max2/1 -> Product3/2
  Constant4/1 -> Max2/2
  Add5/1 -> Unit Delay/1, CACOutletTemp_degC/1
  Add2/1 -> Gain/1
  Gain/1 -> Product2/1  "CACMeanPressure_kPa"
  Product3/1 -> Product2/2
  Product2/1 -> Product4/3  "CACDensity_gpL"
  Constant1/1 -> Product4/1
  Constant6/1 -> Max1/2
  Product4/1 -> Max1/1
  Max1/1 -> Math Function/1
  Math Function/1 -> Product1/4
  Constant7/1 -> Product1/3
  Gain1/1 -> Product4/2
  Constant8/1 -> Product1/1
  Product1/1 -> CACEffectivenessData_frac Table/1, CACMassFlow_gps/1
  Add3/1 -> Gain1/1  "CACDeltaPressure_kPa"
  CompressorOutletPress_kPa/1 -> Add3/1, Add2/1
  Add4/1 -> Product5/1
  Product5/1 -> Add5/2
  CompressorOutletTemp_degC/1 -> Add6/2, Add4/1, Add5/1
  AmbientTemp_degC/1 -> Add4/2
  CACEffectivenessData_frac Table/1 -> Product5/2  "CACEffectiveness_frac"
  Add6/1 -> Gain2/1
  Gain2/1 -> Add1/1  "CACCMeanTemp_degC"
  Unit Delay/1 -> Add6/1

== system EPD629_WilliamsJ_AS12/AirSystemPlantModel/EGRFlow ==
  CoolantTemp_degC : Inport
  EGRValvePositionCmd_pct : Inport  Port=2
  ExhaustManifoldPress_kPa : Inport  Port=3
  ExhaustManifoldTemp_degC : Inport  Port=4
  IntakeManifoldPress_kPa : Inport  Port=5
  EGRCooler : Subsystem
  EGRCoolerOutletPressure : Subsystem
  EGRCoolerOutletTemperature : Subsystem
  EGRValve : Subsystem
  Unit Delay : UnitDelay  InitialCondition=100  SampleTime=-1  HasFrameUpgradeWarning=on
      settings: AttributesFormatString=IC: %<InitialCondition>
  EGRCOutletTemp_degC : Outport
  EGRMassFlow_gps : Outport  Port=2
  wires:
  ExhaustManifoldTemp_degC/1 -> EGRCoolerOutletTemperature/2(ExhaustManifoldTemp_degC), EGRCooler/2(ExhaustManifoldTemp_degC)
  EGRValvePositionCmd_pct/1 -> EGRValve/2(EGRValvePositionCmd_pct)
  CoolantTemp_degC/1 -> EGRCoolerOutletTemperature/3(CoolantTemp_degC)
  EGRCoolerOutletTemperature/1(EGRCOutletTemp_degC) -> EGRCoolerOutletPressure/3(EGRCOutletTemp_degC), Unit Delay/1, EGRCOutletTemp_degC/1
  IntakeManifoldPress_kPa/1 -> EGRValve/1(IntakeManifoldPress_kPa)
  ExhaustManifoldPress_kPa/1 -> EGRCooler/1(ExhaustManifoldPress_kPa)
  EGRValve/1(EGRValveMassFlow_gps) -> EGRCoolerOutletPressure/2(EGRValveMassFlow_gps), EGRCoolerOutletTemperature/1(EGRMassFlow_gps), EGRMassFlow_gps/1
  EGRCooler/1(EGRCoolerMassFlow_gps) -> EGRCoolerOutletPressure/1(EGRCoolerMassFlow_gps)
  Unit Delay/1 -> EGRCooler/4(EGRCOutletTemp_degC), EGRValve/4(EGRCOutletTemp_degC)
  EGRCoolerOutletPressure/1(EGRCOutletPress_kPa) -> EGRCooler/3(EGRCOutletPress_kPa), EGRValve/3(EGRCOutletPress_kPa)

== system EPD629_WilliamsJ_AS12/AirSystemPlantModel/EngineFlow ==
  DesiredFuel_mg : Inport
  EngineSpeed_rpm : Inport  Port=2
  ExhaustManifoldPress_kPa : Inport  Port=3
  IntakeManifoldMassFracO2 : Inport  Port=4
  IntakeManifoldPress_kPa : Inport  Port=5
  IntakeManifoldTemp_degC : Inport  Port=6
  CylinderEVO : Subsystem
  CylinderIVC : Subsystem
  ExhaustTempAndResidualMass : Subsystem
  SpeedDensityMassFlow : Subsystem
  Terminator : Terminator
  Unit Delay : UnitDelay  SampleTime=-1  HasFrameUpgradeWarning=on
      settings: AttributesFormatString=IC: %<InitialCondition>
  Unit Delay1 : UnitDelay  SampleTime=-1  HasFrameUpgradeWarning=on
      settings: AttributesFormatString=IC: %<InitialCondition>
  SpeedDensityMassFlow_gps : Outport
  CylinderIVCMassAir_mg : Outport  Port=2
  CylinderIVCMassFracO2 : Outport  Port=3
  CylindersOutMassFlow_gps : Outport  Port=4
  CylindersOutMassFracO2 : Outport  Port=5
  CylindersOutTemp_degC : Outport  Port=6
  wires:
  CylinderIVC/2(CylinderIVCMassFracO2) -> CylinderIVCMassFracO2/1
  Unit Delay1/1 -> ExhaustTempAndResidualMass/3(CombustionMassFuel_mg)
  CylinderEVO/3(CombustionMassFuel_mg) -> Unit Delay1/1
  Unit Delay/1 -> CylinderIVC/4(CylindersOutMassFracO2)
  CylinderIVC/4(CylinderIVCMass_mg) -> CylinderEVO/2(CylinderIVCMass_mg)
  CylinderEVO/1(CylindersOutMassFlow_gps) -> CylindersOutMassFlow_gps/1
  CylinderEVO/2(CylindersOutMassFracO2) -> CylindersOutMassFracO2/1, Unit Delay/1
  DesiredFuel_mg/1 -> CylinderEVO/5(DesiredFuel_mg)
  CylinderIVC/3(CylinderIVCMassAir_mg) -> CylinderIVCMassAir_mg/1, CylinderEVO/1(CylinderIVCMassAir_mg)
  IntakeManifoldMassFracO2/1 -> CylinderIVC/2(IntakeManifoldMassFracO2)
  SpeedDensityMassFlow/2(CylinderInMass_mg) -> CylinderIVC/1(CylinderInMass_mg)
  ExhaustTempAndResidualMass/1(CylinderResidualMass_mg) -> CylinderEVO/4(CylinderResidualMass_mg), CylinderIVC/3(CylinderResidualMass_mg)
  ExhaustTempAndResidualMass/2(CylindersOutTemp_degC) -> CylindersOutTemp_degC/1
  ExhaustManifoldPress_kPa/1 -> ExhaustTempAndResidualMass/2(ExhaustManifoldPress_kPa)
  IntakeManifoldTemp_degC/1 -> SpeedDensityMassFlow/2(IntakeManifoldTemp_degC)
  IntakeManifoldPress_kPa/1 -> SpeedDensityMassFlow/1(IntakeManifoldPress_kPa)
  EngineSpeed_rpm/1 -> SpeedDensityMassFlow/3(EngineSpeed_rpm), ExhaustTempAndResidualMass/1(EngineSpeed_rpm), CylinderEVO/3(EngineSpeed_rpm)
  SpeedDensityMassFlow/1(SpeedDensityMassFlow_gps) -> SpeedDensityMassFlow_gps/1
  CylinderIVC/1(CylinderResidualMassO2_mg) -> Terminator/1

== system EPD629_WilliamsJ_AS12/AirSystemPlantModel/ExhaustManifold ==
  note: dmO2/dt
  note: dm/dt
  EGRMassFlow_gps : Inport
  CylindersOutMassFlow_gps : Inport  Port=2
  CylindersOutMassFracO2 : Inport  Port=3
  CylindersOutTemp_degC : Inport  Port=4
  TurbineMassFlow_gps : Inport  Port=5
  WastegateMassFlow_gps : Inport  Port=6
  Add : Sum  Inputs=+-
  Add1 : Sum  Inputs=3
  Add2 : Sum  Inputs=+-
  Add7 : Sum
  Constant7 : Constant  Value=273.15
  Constant8 : Constant  Value=ExhaustManifoldGasConstant_kJpkgK
  Constant9 : Constant  Value=ExhaustManifoldVolume_L
  Integrator1 : Integrator  LimitOutput=on  UpperSaturationLimit=1000  LowerSaturationLimit=0
      settings: AttributesFormatString=|
      | Max: %<UpperSaturationLimit>
      | Min: %<LowerSaturationLimit>
      | IC: %<InitialCondition>
  Integrator3 : Integrator  InitialCondition=10  LimitOutput=on  UpperSaturationLimit=1000  LowerSaturationLimit=1
      settings: AttributesFormatString=|
      | Max: %<UpperSaturationLimit>
      | Min: %<LowerSaturationLimit>
      | IC: %<InitialCondition>
  Product1 : Product  RndMeth=Zero
  Product11 : Product  Inputs=**/  RndMeth=Zero
  Product4 : Product  RndMeth=Zero
  Product6 : Product  RndMeth=Zero
  Product7 : Product  Inputs=*/  RndMeth=Zero
  Saturation : Saturate  UpperLimit=1000  LowerLimit=-100
      settings: AttributesFormatString=|
      | Max: %<UpperLimit>
      | Min: %<LowerLimit>
  Transfer Fcn : TransferFcn  Denominator=[0.05 1]
  ExhaustManifoldMassFracO2 : Outport
  ExhaustManifoldPress_kPa : Outport  Port=2
  ExhaustManifoldTemp_degC : Outport  Port=3
  wires:
  Integrator1/1 -> Product7/1  "ExhaustManifoldMassO2_g"
  Add2/1 -> Integrator1/1
  Product11/1 -> Product1/2
  Constant8/1 -> Product11/1
  Add7/1 -> Product11/2
  Constant9/1 -> Product11/3
  Add/1 -> Integrator3/1
  Constant7/1 -> Add7/2
  Product7/1 -> ExhaustManifoldMassFracO2/1, Product6/2
  Saturation/1 -> Transfer Fcn/1
  Product6/1 -> Add2/2
  Product4/1 -> Add2/1
  CylindersOutMassFracO2/1 -> Product4/2
  CylindersOutTemp_degC/1 -> Saturation/1
  EGRMassFlow_gps/1 -> Add1/1
  TurbineMassFlow_gps/1 -> Add1/2
  WastegateMassFlow_gps/1 -> Add1/3
  Add1/1 -> Product6/1, Add/2
  Integrator3/1 -> Product1/1, Product7/2
  Product1/1 -> ExhaustManifoldPress_kPa/1
  Transfer Fcn/1 -> ExhaustManifoldTemp_degC/1, Add7/1
  CylindersOutMassFlow_gps/1 -> Product4/1, Add/1

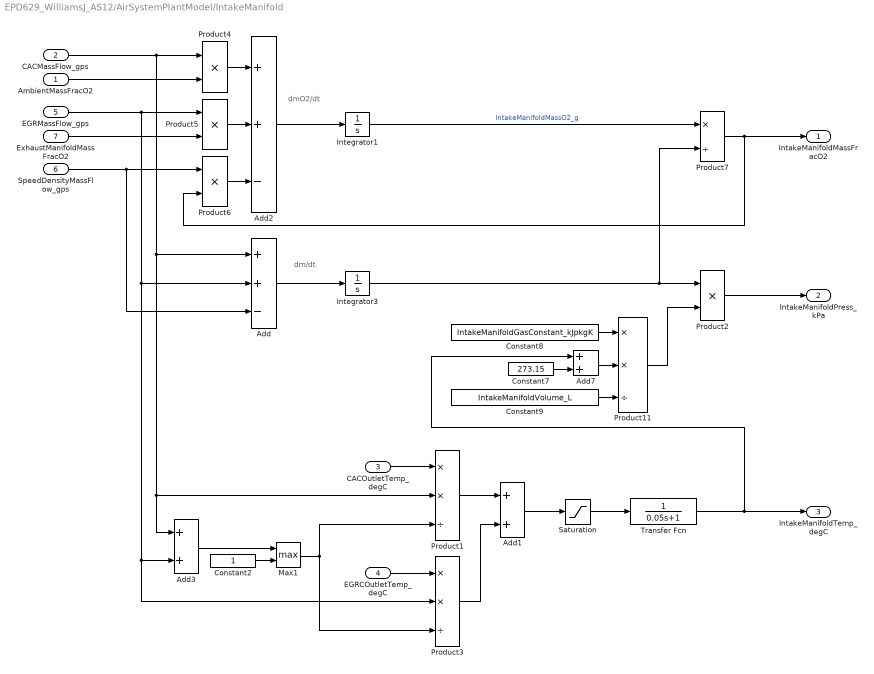
== system EPD629_WilliamsJ_AS12/AirSystemPlantModel/IntakeManifold ==
  note: dm/dt
  note: dmO2/dt
  AmbientMassFracO2 : Inport
  CACMassFlow_gps : Inport  Port=2
  CACOutletTemp_degC : Inport  Port=3
  EGRCOutletTemp_degC : Inport  Port=4
  EGRMassFlow_gps : Inport  Port=5
  SpeedDensityMassFlow_gps : Inport  Port=6
  ExhaustManifoldMassFracO2 : Inport  Port=7
  Add : Sum  Inputs=++-
  Add1 : Sum  Inputs=2
  Add2 : Sum  Inputs=++-
  Add3 : Sum  Inputs=2
  Add7 : Sum
  Constant2 : Constant
  Constant7 : Constant  Value=273.15
  Constant8 : Constant  Value=IntakeManifoldGasConstant_kJpkgK
  Constant9 : Constant  Value=IntakeManifoldVolume_L
  Integrator1 : Integrator  LimitOutput=on  UpperSaturationLimit=1000  LowerSaturationLimit=0
      settings: AttributesFormatString=|
      | Max: %<UpperSaturationLimit>
      | Min: %<LowerSaturationLimit>
      | IC: %<InitialCondition>
  Integrator3 : Integrator  InitialCondition=10  LimitOutput=on  UpperSaturationLimit=1000  LowerSaturationLimit=1
      settings: AttributesFormatString=|
      | Max: %<UpperSaturationLimit>
      | Min: %<LowerSaturationLimit>
      | IC: %<InitialCondition>
  Max1 : MinMax  Function=max  Inputs=2
  Product1 : Product  Inputs=**/  RndMeth=Zero
  Product11 : Product  Inputs=**/  RndMeth=Zero
  Product{2,4..6} (4 alike) : Product  RndMeth=Zero
  Product3 : Product  Inputs=**/  RndMeth=Zero
  Product7 : Product  Inputs=*/  RndMeth=Zero
  Saturation : Saturate  UpperLimit=1000  LowerLimit=-100
      settings: AttributesFormatString=|
      | Max: %<UpperLimit>
      | Min: %<LowerLimit>
  Transfer Fcn : TransferFcn  Denominator=[0.05 1]
  IntakeManifoldMassFracO2 : Outport
  IntakeManifoldPress_kPa : Outport  Port=2
  IntakeManifoldTemp_degC : Outport  Port=3
  wires:
  CACMassFlow_gps/1 -> Add3/1, Product1/2, Add/1, Product4/1
  SpeedDensityMassFlow_gps/1 -> Product6/1, Add/3
  CACOutletTemp_degC/1 -> Product1/1
  EGRCOutletTemp_degC/1 -> Product3/1
  Constant2/1 -> Max1/2
  Add3/1 -> Max1/1
  Max1/1 -> Product1/3, Product3/3
  EGRMassFlow_gps/1 -> Product3/2, Add3/2, Add/2, Product5/1
  Product1/1 -> Add1/1
  Product3/1 -> Add1/2
  Product4/1 -> Add2/1
  Product5/1 -> Add2/2
  Product6/1 -> Add2/3
  Add1/1 -> Saturation/1
  Saturation/1 -> Transfer Fcn/1
  Product7/1 -> IntakeManifoldMassFracO2/1, Product6/2
  Constant7/1 -> Add7/2
  Constant9/1 -> Product11/3
  Add7/1 -> Product11/2
  Constant8/1 -> Product11/1
  Add2/1 -> Integrator1/1
  Integrator1/1 -> Product7/1  "IntakeManifoldMassO2_g"
  AmbientMassFracO2/1 -> Product4/2
  ExhaustManifoldMassFracO2/1 -> Product5/2
  Integrator3/1 -> Product7/2, Product2/1
  Product11/1 -> Product2/2
  Add/1 -> Integrator3/1
  Product2/1 -> IntakeManifoldPress_kPa/1
  Transfer Fcn/1 -> Add7/1, IntakeManifoldTemp_degC/1

== system EPD629_WilliamsJ_AS12/AirSystemPlantModel/TurbineOutletPressure ==
  note: dP/dt
  note: dm/dt
  TurbineMassFlow_gps : Inport
  TurbineOutletTemp_degC : Inport  Port=2
  WastegateMassFlow_gps : Inport  Port=3
  BPVFlow_gps : Inport  Port=4
  ExhaustManifoldTemp_degC : Inport  Port=5
  Add : Sum  Inputs=++-
  Add1 : Sum  Inputs=2
  Add3 : Sum  Inputs=2
  Add7 : Sum
  Constant2 : Constant
  Constant7 : Constant  Value=273.15
  Constant8 : Constant  Value=ExhaustManifoldGasConstant_kJpkgK
  Constant9 : Constant  Value=TurbineToBPVVolume_L
  Integrator3 : Integrator  InitialCondition=100  LimitOutput=on  UpperSaturationLimit=1000  LowerSaturationLimit=10
      settings: AttributesFormatString=|
      | Max: %<UpperSaturationLimit>
      | Min: %<LowerSaturationLimit>
      | IC: %<InitialCondition>
  Max1 : MinMax  Function=max  Inputs=2
  Product1 : Product  Inputs=**/  RndMeth=Zero
  Product11 : Product  Inputs=**/  RndMeth=Zero
  Product2 : Product  RndMeth=Zero
  Product3 : Product  Inputs=**/  RndMeth=Zero
  Saturation : Saturate  UpperLimit=1000  LowerLimit=-100
      settings: AttributesFormatString=|
      | Max: %<UpperLimit>
      | Min: %<LowerLimit>
  Transfer Fcn : TransferFcn  Denominator=[0.05 1]
  BPVInletTemp_degC : Outport
  TurbineOutletPress_kPa : Outport  Port=2
  wires:
  Product2/1 -> Integrator3/1
  Product11/1 -> Product2/2
  Constant8/1 -> Product11/1
  Add7/1 -> Product11/2
  Constant9/1 -> Product11/3
  Add/1 -> Product2/1
  Constant7/1 -> Add7/2
  Saturation/1 -> Transfer Fcn/1
  Add1/1 -> Saturation/1
  Product3/1 -> Add1/2
  Product1/1 -> Add1/1
  WastegateMassFlow_gps/1 -> Add/2, Add3/2, Product3/2
  Max1/1 -> Product3/3, Product1/3
  Add3/1 -> Max1/1
  Constant2/1 -> Max1/2
  ExhaustManifoldTemp_degC/1 -> Product3/1
  TurbineOutletTemp_degC/1 -> Product1/1
  BPVFlow_gps/1 -> Add/3
  TurbineMassFlow_gps/1 -> Add/1, Product1/2, Add3/1
  Integrator3/1 -> TurbineOutletPress_kPa/1
  Transfer Fcn/1 -> Add7/1, BPVInletTemp_degC/1

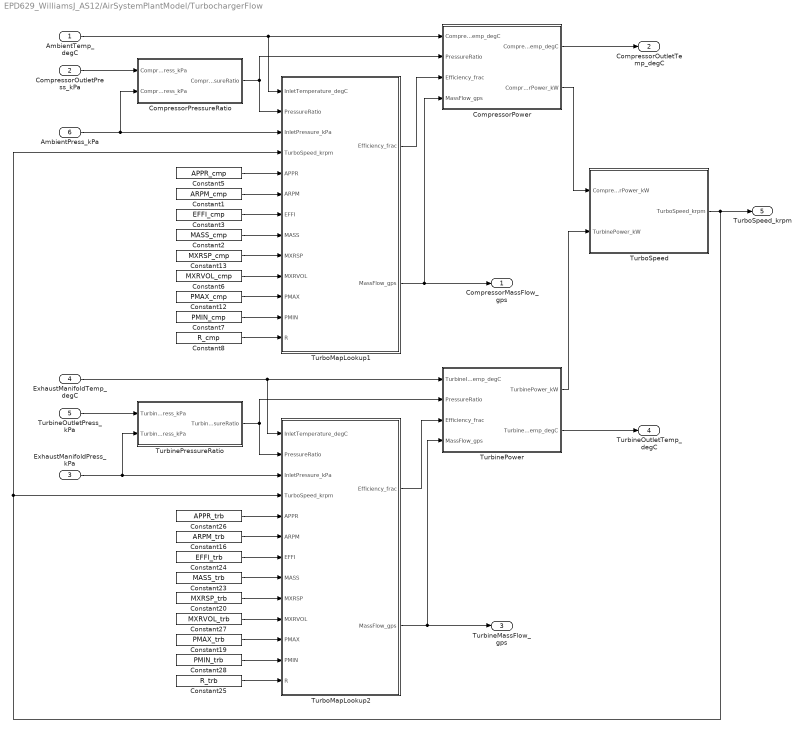
== system EPD629_WilliamsJ_AS12/AirSystemPlantModel/TurbochargerFlow ==
  AmbientTemp_degC : Inport
  CompressorOutletPress_kPa : Inport  Port=2
  ExhaustManifoldPress_kPa : Inport  Port=3
  ExhaustManifoldTemp_degC : Inport  Port=4
  TurbineOutletPress_kPa : Inport  Port=5
  AmbientPress_kPa : Inport  Port=6
  CompressorPower : Subsystem
  CompressorPressureRatio : Subsystem
  Constant1 : Constant  Value=ARPM_cmp
  Constant12 : Constant  Value=PMAX_cmp
  Constant13 : Constant  Value=MXRSP_cmp
  Constant16 : Constant  Value=ARPM_trb
  Constant19 : Constant  Value=PMAX_trb
  Constant2 : Constant  Value=MASS_cmp
  Constant20 : Constant  Value=MXRSP_trb
  Constant23 : Constant  Value=MASS_trb
  Constant24 : Constant  Value=EFFI_trb
  Constant25 : Constant  Value=R_trb
  Constant26 : Constant  Value=APPR_trb
  Constant27 : Constant  Value=MXRVOL_trb
  Constant28 : Constant  Value=PMIN_trb
  Constant3 : Constant  Value=EFFI_cmp
  Constant5 : Constant  Value=APPR_cmp
  Constant6 : Constant  Value=MXRVOL_cmp
  Constant7 : Constant  Value=PMIN_cmp
  Constant8 : Constant  Value=R_cmp
  TurbinePower : Subsystem
  TurbinePressureRatio : Subsystem
  TurboMapLookup1 : Subsystem
  TurboMapLookup2 : Subsystem
  TurboSpeed : Subsystem
  CompressorMassFlow_gps : Outport
  CompressorOutletTemp_degC : Outport  Port=2
  TurbineMassFlow_gps : Outport  Port=3
  TurbineOutletTemp_degC : Outport  Port=4
  TurboSpeed_krpm : Outport  Port=5
  wires:
  AmbientTemp_degC/1 -> TurboMapLookup1/1(InletTemperature_degC), CompressorPower/1(CompressorInletTemp_degC)
  TurboSpeed/1(TurboSpeed_krpm) -> TurboSpeed_krpm/1, TurboMapLookup2/4(TurboSpeed_krpm), TurboMapLookup1/4(TurboSpeed_krpm)
  Constant12/1 -> TurboMapLookup1/11(PMAX)
  Constant23/1 -> TurboMapLookup2/8(MASS)
  Constant1/1 -> TurboMapLookup1/6(ARPM)
  TurboMapLookup2/2(MassFlow_gps) -> TurbineMassFlow_gps/1, TurbinePower/4(MassFlow_gps)
  TurbinePressureRatio/1(TurbinePressureRatio) -> TurbinePower/2(PressureRatio), TurboMapLookup2/2(PressureRatio)
  CompressorPressureRatio/1(CompressorPressureRatio) -> TurboMapLookup1/2(PressureRatio), CompressorPower/2(PressureRatio)
  Constant7/1 -> TurboMapLookup1/12(PMIN)
  Constant2/1 -> TurboMapLookup1/8(MASS)
  TurboMapLookup1/1(Efficiency_frac) -> CompressorPower/3(Efficiency_frac)
  Constant6/1 -> TurboMapLookup1/10(MXRVOL)
  Constant5/1 -> TurboMapLookup1/5(APPR)
  ExhaustManifoldTemp_degC/1 -> TurboMapLookup2/1(InletTemperature_degC), TurbinePower/1(TurbineInletTemp_degC)
  Constant13/1 -> TurboMapLookup1/9(MXRSP)
  Constant20/1 -> TurboMapLookup2/9(MXRSP)
  CompressorPower/2(CompressorPower_kW) -> TurboSpeed/1(CompressorPower_kW)
  Constant24/1 -> TurboMapLookup2/7(EFFI)
  TurboMapLookup1/2(MassFlow_gps) -> CompressorPower/4(MassFlow_gps), CompressorMassFlow_gps/1
  TurbinePower/1(TurbinePower_kW) -> TurboSpeed/2(TurbinePower_kW)
  Constant26/1 -> TurboMapLookup2/5(APPR)
  Constant28/1 -> TurboMapLookup2/12(PMIN)
  Constant25/1 -> TurboMapLookup2/13(R)
  Constant8/1 -> TurboMapLookup1/13(R)
  Constant19/1 -> TurboMapLookup2/11(PMAX)
  TurboMapLookup2/1(Efficiency_frac) -> TurbinePower/3(Efficiency_frac)
  Constant3/1 -> TurboMapLookup1/7(EFFI)
  Constant16/1 -> TurboMapLookup2/6(ARPM)
  Constant27/1 -> TurboMapLookup2/10(MXRVOL)
  AmbientPress_kPa/1 -> CompressorPressureRatio/2(CompressorInletPress_kPa), TurboMapLookup1/3(InletPressure_kPa)
  ExhaustManifoldPress_kPa/1 -> TurbinePressureRatio/2(TurbineInletPress_kPa), TurboMapLookup2/3(InletPressure_kPa)
  CompressorPower/1(CompressorOutletTemp_degC) -> CompressorOutletTemp_degC/1
  TurbinePower/2(TurbineOutletTemp_degC) -> TurbineOutletTemp_degC/1
  CompressorOutletPress_kPa/1 -> CompressorPressureRatio/1(CompressorOutletPress_kPa)
  TurbineOutletPress_kPa/1 -> TurbinePressureRatio/1(TurbineOutletPress_kPa)

== system EPD629_WilliamsJ_AS12/AirSystemPlantModel/WastegateFlow ==
  note: kPa
  note: m/s
  note: N*m/kg
  note: k kg*m/s^2/m^2
  note: m^2/s^2
  note: g*m/s^2/mm^2
  note: K
  AmbientPress_kPa : Inport
  TurbineOutletPress_kPa : Inport  Port=2
  CompressorOutletPress_kPa : Inport  Port=3
  ExhaustManifoldPress_kPa : Inport  Port=4
  ExhaustManifoldTemp_degC : Inport  Port=5
  Add : Sum  Inputs=+-
  Add1 : Sum
  Constant : Constant  Value=273.15
  Constant1 : Constant  Value=DischargeCoefficient_frac
  Constant2 : Constant
  Constant3 : Constant  Value=ExhaustManifoldGasConstant_kJpkgK
  Constant5 : Constant  Value=WastegateWideOpenArea_mm2
  Constant6 : Constant  Value=100
  FlowFunctionData_frac Table : Lookup_n-D  NumberOfTableDimensions=1  BreakpointsForDimension1=PressureRatioBreakpoints_frac  Table=FlowFunctionData_frac  ExtrapMethod=Clip  UseLastTableValue=on  InternalRulePriority=Speed  RndMeth=Simplest  InputSameDT=on
  Math Function : Math  Operator=sqrt  SignedPower=on  SaturateOnIntegerOverflow=on
  Max2 : MinMax  Function=max  Inputs=2
  Product : Product  Inputs=**/
  Product1 : Product  Inputs=****/  SaturateOnIntegerOverflow=on  OutDataTypeStr=Inherit: Same as first input
  Product2 : Product  Inputs=*/  SaturateOnIntegerOverflow=on  OutDataTypeStr=Inherit: Same as first input
  Product3 : Product  SaturateOnIntegerOverflow=on  OutDataTypeStr=Inherit: Same as first input
  WastegateAreaData_pct Table : Lookup_n-D  NumberOfTableDimensions=1  BreakpointsForDimension1=WastegateAreaGagePressBreakpoints_kPa  Table=WastegateAreaData_pct  ExtrapMethod=Clip  UseLastTableValue=on  InternalRulePriority=Speed  RndMeth=Simplest  InputSameDT=on
  kJ/(kg*K) to J/(kg*K) : Gain  Gain=1000
  WastegateMassFlow_gps : Outport
  wires:
  TurbineOutletPress_kPa/1 -> Product2/1
  Product1/1 -> WastegateMassFlow_gps/1
  ExhaustManifoldPress_kPa/1 -> Product1/4, Product2/2
  WastegateAreaData_pct Table/1 -> Product/1  "WastegateArea_pct"
  FlowFunctionData_frac Table/1 -> Product1/3
  Product2/1 -> FlowFunctionData_frac Table/1  "WastegatePressureRatio_frac"
  Constant1/1 -> Product1/2
  Constant3/1 -> kJ/(kg*K) to J/(kg*K)/1
  kJ/(kg*K) to J/(kg*K)/1 -> Product3/1
  Max2/1 -> Product3/2
  Math Function/1 -> Product1/5
  Product3/1 -> Math Function/1
  Constant6/1 -> Product/3
  Constant5/1 -> Product/2
  Product/1 -> Product1/1  "WastegateArea_mm2"
  CompressorOutletPress_kPa/1 -> Add/1
  AmbientPress_kPa/1 -> Add/2
  Add/1 -> WastegateAreaData_pct Table/1
  ExhaustManifoldTemp_degC/1 -> Add1/1
  Constant2/1 -> Max2/2
  Constant/1 -> Add1/2
  Add1/1 -> Max2/1

== system EPD629_WilliamsJ_AS12/EGRFlowControl/CoolerOutletPressureCommand ==
  ExhaustManifoldPressSens_kPa : Inport
  ExhaustManifoldTempEst_degC : Inport  Port=2
  EGRCOutletTempSens_degC : Inport  Port=3
  EGRMassFlowCmd_gps : Inport  Port=4
  Add : Sum
  Add1 : Sum
  Constant : Constant  Value=.001
  Constant1 : Constant  Value=EGRCFlowRestrictionArea_mm2
  Constant2 : Constant  Value=EGRCDischargeCoefficient_frac
  Constant3 : Constant  Value=0.5
  Constant4 : Constant  Value=273.15
  Constant5 : Constant  Value=ExhaustManifoldGasConstant_kJpkgK
  Constant6 : Constant
  Constant7 : Constant  Value=.001
  Divide : Product  Inputs=*/
  Divide1 : Product  Inputs=**/
  Divide2 : Product  Inputs=*/
  Gain : Gain  Gain=.001
  Gain1 : Gain  Gain=0.5
  Max : MinMax  Function=max  Inputs=2
  Max1 : MinMax  Function=max  Inputs=2
  Product : Product  Inputs=3
  Product1 : Product
  Square : Math  Operator=square  SaturateOnIntegerOverflow=on
  Subtract : Sum  Inputs=+-
  EGRCOutletPressCmd_kPa : Outport
  wires:
  ExhaustManifoldPressSens_kPa/1 -> Divide2/1, Subtract/1
  EGRMassFlowCmd_gps/1 -> Divide/1
  Constant/1 -> Product/1
  Constant1/1 -> Product/2
  Constant2/1 -> Product/3
  Product/1 -> Divide/2
  Divide/1 -> Square/1
  Square/1 -> Divide1/2
  Constant3/1 -> Divide1/1
  Divide1/1 -> Gain/1
  Gain/1 -> Subtract/2  "EGRCDeltaPressCmd (kPa)"
  Subtract/1 -> EGRCOutletPressCmd_kPa/1
  ExhaustManifoldTempEst_degC/1 -> Add/1
  EGRCOutletTempSens_degC/1 -> Add/2
  Add/1 -> Gain1/1
  Gain1/1 -> Add1/1  "EGRCMeanTemp (C)"
  Constant4/1 -> Add1/2
  Max/1 -> Product1/2
  Add1/1 -> Max/1
  Constant6/1 -> Max/2
  Constant5/1 -> Product1/1
  Product1/1 -> Divide2/2
  Constant7/1 -> Max1/2
  Divide2/1 -> Max1/1  "g/L (kg/m3)"
  Max1/1 -> Divide1/3  "EGR Cooler Density (gpl)"
